simulink model "Speedtest"  (R2018a)
settings: Solver=ode4  StartTime=0.0  StopTime=100  FixedStep=0.08  RelTol=1e-3
libraries: simulink x2
settings Model: Creator=Hungs  LastModifiedBy=Hungs

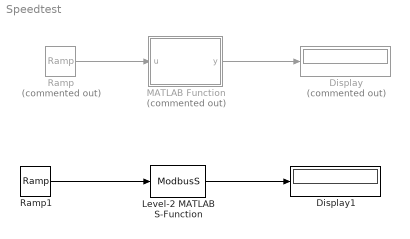
== system Speedtest ==
  Display : Display  Commented=on
  Display1 : Display
  Level-2 MATLAB S-Function : M-S-Function  FunctionName=ModbusS
  MATLAB Function : MATLAB Function  Commented=on  TreatAsAtomicUnit=on
  Ramp : simulink/Sources/Ramp  Commented=on  slope=1  start=0  InitialOutput=0
  Ramp1 : simulink/Sources/Ramp  slope=1  start=0  InitialOutput=0
  wires:
  Ramp/1 -> MATLAB Function/1(u)
  MATLAB Function/1(y) -> Display/1
  Ramp1/1 -> Level-2 MATLAB S-Function/1
  Level-2 MATLAB S-Function/1 -> Display1/1

== matlab function Speedtest/MATLAB Function ==
  data: u input; y output
function y = fcn(u)
    a = 0;
    coder.extrinsic('modbus');
    coder.extrinsic('read');
    coder.extrinsic('write');
    m = modbus('tcpip', '127.0.0.1', 502);
    a = (read(m,'holdingregs',100,1,'double'));
    write(m,'holdingregs',100,u,'double');
y = a;
